simulink model "DriveSimulation"  (R2019b)
settings: Solver=FixedStepAuto  StartTime=0.0  StopTime=inf  FixedStep=dt  RelTol=1e-3
model workspace (MAT data in the model file):
  AcceNoisePower = 0.01
  AcceNoiseStd = 0.1
  AcceTs = 0.01
  ControlTs = 0.1
  GPSNoisePower = 0.001
  GPSNoiseStd = 1
  GPSTs = 0.5
  GyroNoisePower = 0.001
  GyroNoiseStd = 0.000174532925199
  GyroTs = 0.01
  L = 4
  SteeringRange = 0.837758040957
  Ts = 0.01
  Var = 0
  Vmax = 41.6666666667
  dt = 0.01
undefined symbols (not defined in the file): DiscIntNeverNeededParam, m, rad, s
libraries: simulink x6, sim3dlib x1, sim3dautolib x1, aerolibanimutils x1
settings Model: Creator=alons  LastModifiedBy=alons
settings DataIOCC: ReturnWorkspaceOutputs=off
settings DebuggingCC: ArithmeticOperatorsInVariantConditions=warning
settings SFSimCC: CustomCodeUndefinedFunction=UseInterfaceOnly

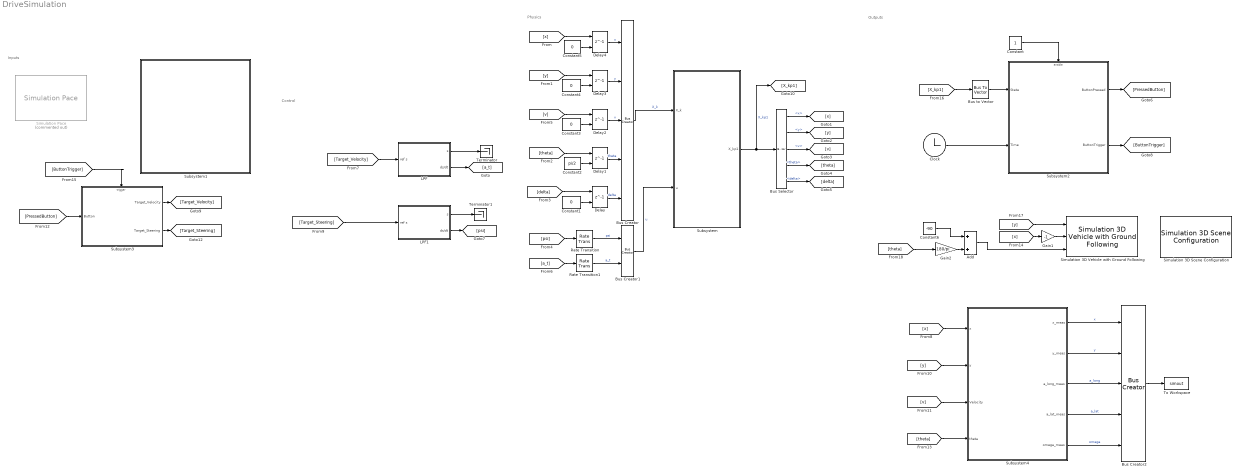
== system DriveSimulation ==
  note: Control
  note: Physics
  note: Inputs
  note: Outputs
  Add : Sum
  Bus Creator : BusCreator  Inputs=5
  Bus Creator1 : BusCreator  Inputs=2
  Bus Creator2 : BusCreator  Inputs=5
  Bus Selector : BusSelector  OutputSignals=x,y,v,theta,delta
  Bus to Vector : BusToVector
  Clock : Clock
  Constant : Constant  SampleTime=0
      settings: OpenFcn=|
      | if get_param(gcbh,'value')-48
      |    set_param(gcbh,'value','0','backgroundcolor','red');
      | else
      |    set_param(gcbh,'value','1','backgroundcolor','green');
      | end
  Constant{1,3..5} (4 alike) : Constant  Value=0
  Constant2 : Constant  Value=pi/2
  Constant6 : Constant  Value=-90
  Delay{,1..4} (5 alike) : Delay  DelayLength=1  InitialConditionSource=Input port
      settings: InputPortMap=u0,p4
  Gain1 : Gain  Gain=-1
  Gain2 : Gain  Gain=180/pi
  LPF : Subsystem  mask{Freq=1, Rate_Max=10 %m/s^2, Rate_Min=-20 %m/s^2}
      mask prompts: Freq "LPF Freq [Hz]"; Rate_Max "Maximum ds/dt slope"; Rate_Min "Minimum ds/dt slope"
      mask Display: fprintf('LPF /w Rate Limit \n%g[Hz]',Freq);
  LPF1 : Subsystem  mask{Freq=2, Rate_Max=20*pi/180 %rad/s, Rate_Min=-20*pi/180 %rad/s}
      mask prompts: Freq "LPF Freq [Hz]"; Rate_Max "Maximum ds/dt slope"; Rate_Min "Minimum ds/dt slope"
      mask Display: fprintf('LPF /w Rate Limit \n%g[Hz]',Freq);
  Rate Transition : RateTransition  OutPortSampleTime=dt
  Rate Transition1 : RateTransition  OutPortSampleTime=dt
  Simulation 3D Scene Configuration : sim3dlib/Simulation 3D Scene Configuration  Priority=0  SceneDesc=Curved road  vehTagList={'Scene Origin';'SimulinkVehicle1'}  vehTag=SimulinkVehicle1  OpVisEn=off  Ts=ControlTs  ProjectFormat=Executable  ProjectName=VehicleSimulation.exe  sensorTag=MainCamera1  sensorId=1  sensorName=MainCamera1  mountLoc=Origin  offsetFlag=off  tmountOffset=[0, 0, 0]  rmountOffset=[0, 0, 0]  HorizontalResolution=1280  VerticalResolution=720  HorizontalFOV=60  mountPoint=[0 0 0]  mountOrientation=[0 0 0]  aMode=3  ID=1
      settings: SourceProductName=Automated Driving Toolbox  SourceProductBaseCode=DR
  Simulation 3D Vehicle with Ground Following : sim3dautolib/Simulation 3D Vehicle with Ground Following  Priority=-1  PassVehMesh=Muscle car  VehColor=Red  InitialPos=[0, 0, 0]  InitialRot=[0, 0, 0]  ActorName=SimulinkVehicle1  SampleTime=-1  ActorType=SimulinkVehicle  ID=1  aMode=3  ActorTag=SimulinkVehicle1  CoordinateScheme=ISO  TransformOutportEnabled=off
      settings: SourceProductName=Automated Driving Toolbox  SourceProductBaseCode=DR
  Simulation Pace : aerolibanimutils/Simulation Pace  Commented=on  SimulationPace=1  SleepMode=Auto  OutputPaceError=off  SampleTime=dt
  Subsystem : Subsystem
      mask Display: fprintf('Rear Axle Bicycle Model\n[Kinematic]')
  Subsystem1 : Subsystem  InitFcn=|  mask{dt=0.01, ControlTs=0.1, AcceTs=0.01, GyroTs=0.01, GPSTs=0.5, AcceNoiseStd=0.1, GyroNoiseStd=0.01*pi/180, GPSNoiseStd=1, L=4, Vmax=150/3.6, SteeringRange=48/180*pi}
      | mdlWks=get_param(bdroot,'ModelWorkspace')
      | par = get_param(gcb,'DialogParameters');
      | fnames = fieldnames(par);
      | for ipar=1:length(fnames)
      |    num=str2num(get_param(gcb,fnames{ipar}));
      |    mdlWks.assignin(fnames{ipar},num);
      | end
      | 
      | clear par fnames ipar num mdlWks;
      mask prompts: dt "Physics Time Sample [s]"; ControlTs "Control Time Sample [s]"; AcceTs "Accelerometer Time Sample [s]"; GyroTs "Gyro Time Sample [s]"; GPSTs "GPS Time Sample [s]"; AcceNoiseStd "Accelerometer Noise std [m/s^2]"; GyroNoiseStd "Gyro Noise std [rad/s]"; GPSNoiseStd "GPS Noise std [m]"; L "Bicycle Length [m]"; Vmax "Maximum Velocity [m/s]"; SteeringRange "Steering Range [rad]"
      mask Display:
      | str=[
      |     'Model Workspace Parameters \n\n\n',...
      |     'Physics Sample dt = %g[s]\n\n',...
      |     'Control Sample ControlTs = %g[s]\n\n',...
      |     'Accelerometer Sample AcceTs = %g[s]\n\n',...
      |     'Gyro Sample GyroTs = %g[s]\n\n',...
      |     'GPS Sample GpsTs = %g[s]\n\n',...
      |     'Accelerometer Noise std = %g[m/s^2]\n\n',...
      |     'Gyro Noise std = %g[rad/s^2]\n\n',...
      |     'GPS Noise std = %g[m]\n\n',...
      |     'Bicycle Length L = %g[m]\n\n',...
      |     'Maximum Velocity Vmax = %g[m/s]\n\n',...
      |     'SteeringRange = %g[rad]\n\n',...
      |     ];
      | fprintf(str,dt,ControlTs,AcceTs,GyroTs,GPSTs,...
      |     AcceNoiseStd,GyroNoiseStd,GPSNoiseStd,L,Vmax,SteeringRange);
  Subsystem2 : Subsystem
      settings: OpenFcn=|
      | UserData = get_param([gcb,'/AnimationSfcn'],'UserData');
      | Fig = UserData.Figure;
      | if ishghandle(Fig,'figure');
      |    %bring to the front:
      |    figure(Fig);
      | end
      mask Display:
      | t=linspace(0,2*pi,20);
      | plot(cos(t),sin(t));
      | 
      | x=[-0.4,-0.4,0.6,-0.4];
      | y=[-0.5,0.5,0,-0.5];
      | plot(x,y)
      | 
      | disp('Drive Simulator')
  Subsystem3 : Subsystem
  Subsystem4 : Subsystem
      mask Display: disp('Sensor Readings')
  Terminator : Terminator
  Terminator1 : Terminator
  To Workspace : ToWorkspace  VariableName=simout  SaveFormat=Timeseries  SampleTime=-1
  wires:
  [psi] -> Rate Transition/1
  [a_t] -> Rate Transition1/1
  Bus Creator/1 -> Subsystem/1(X_k)  "X_k"
  Bus Creator1/1 -> Subsystem/2(u)  "u"
  Constant/1 -> Subsystem2/Enable
  Clock/1 -> Subsystem2/2(Time)
  Bus Selector/2 -> [y]  "<y>"
  Bus Selector/1 -> [x]  "<x>"
  Bus Selector/3 -> [v]  "<v>"
  Bus Selector/5 -> [delta]  "<delta>"
  Bus Selector/4 -> [theta]  "<theta>"
  [Target_Velocity] -> LPF/1(ref s)
  [Target_Steering] -> LPF1/1(ref s)
  LPF1/2(ds/dt) -> [psi]
  [PressedButton] -> Subsystem3/1(Button)
  [ButtonTrigger] -> Subsystem3/Trigger
  Subsystem3/1(Target_Velocity) -> [Target_Velocity]
  Subsystem3/2(Target_Steering) -> [Target_Steering]
  Rate Transition/1 -> Bus Creator1/1  "psi"
  Rate Transition1/1 -> Bus Creator1/2  "a_t"
  [X_kp1] -> Bus to Vector/1
  Bus to Vector/1 -> Subsystem2/1(State)
  Delay/1 -> Bus Creator/5  "delta"
  [delta] -> Delay/1
  Constant1/1 -> Delay/2
  Delay1/1 -> Bus Creator/4  "theta"
  Delay2/1 -> Bus Creator/3  "v"
  Delay3/1 -> Bus Creator/2  "y"
  Delay4/1 -> Bus Creator/1  "x"
  [x] -> Delay4/1
  [v] -> Delay2/1
  [y] -> Delay3/1
  [theta] -> Delay1/1
  Constant2/1 -> Delay1/2
  Constant3/1 -> Delay2/2
  Constant4/1 -> Delay3/2
  Constant5/1 -> Delay4/2
  Subsystem/1(X_kp1) -> [X_kp1], Bus Selector/1  "X_kp1"
  LPF/2(ds/dt) -> [a_t]
  LPF/1(s) -> Terminator/1
  LPF1/1(s) -> Terminator1/1
  Subsystem2/1(ButtonPressed) -> [PressedButton]
  Subsystem2/2(ButtonTrigger) -> [ButtonTrigger]
  [x] -> Subsystem4/1(x)
  [y] -> Subsystem4/2(y)
  [v] -> Subsystem4/3(Velocity)
  [theta] -> Subsystem4/4(theta)
  Subsystem4/5(omega_meas) -> Bus Creator2/5  "omega"
  Subsystem4/4(a_lat_meas) -> Bus Creator2/4  "a_lat"
  Subsystem4/3(a_long_meas) -> Bus Creator2/3  "a_long"
  Subsystem4/2(y_meas) -> Bus Creator2/2  "y"
  Subsystem4/1(x_meas) -> Bus Creator2/1  "x"
  Bus Creator2/1 -> To Workspace/1
  [x] -> Gain1/1
  [theta] -> Gain2/1
  Gain1/1 -> Simulation 3D Vehicle with Ground Following/2
  Gain2/1 -> Add/2
  Add/1 -> Simulation 3D Vehicle with Ground Following/3
  Constant6/1 -> Add/1
  [y] -> Simulation 3D Vehicle with Ground Following/1

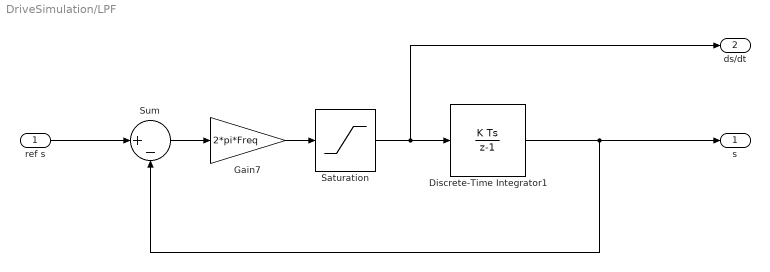
== system DriveSimulation/LPF ==
  ref s : Inport
  Discrete-Time Integrator1 : DiscreteIntegrator  SampleTime=-1  ICPrevOutput=DiscIntNeverNeededParam  ICPrevScaledInput=DiscIntNeverNeededParam
  Gain7 : Gain  Gain=2*pi*Freq
  Saturation : Saturate  UpperLimit=Rate_Max  LowerLimit=Rate_Min
  Sum : Sum  Inputs=|+-
  s : Outport  VectorParamsAs1DForOutWhenUnconnected=off
  ds/dt : Outport  Port=2  VectorParamsAs1DForOutWhenUnconnected=off
  wires:
  Discrete-Time Integrator1/1 -> s/1, Sum/2
  Sum/1 -> Gain7/1
  Gain7/1 -> Saturation/1
  ref s/1 -> Sum/1
  Saturation/1 -> ds/dt/1, Discrete-Time Integrator1/1

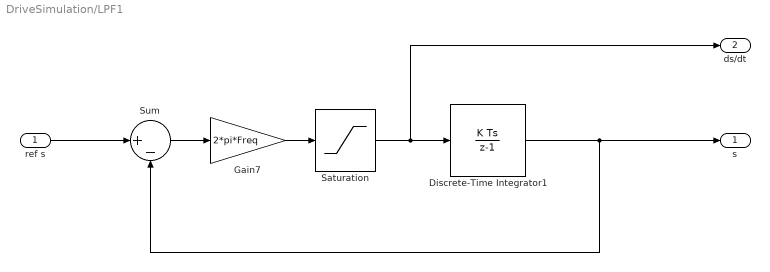
== system DriveSimulation/LPF1 ==
  ref s : Inport
  Discrete-Time Integrator1 : DiscreteIntegrator  SampleTime=-1  ICPrevOutput=DiscIntNeverNeededParam  ICPrevScaledInput=DiscIntNeverNeededParam
  Gain7 : Gain  Gain=2*pi*Freq
  Saturation : Saturate  UpperLimit=Rate_Max  LowerLimit=Rate_Min
  Sum : Sum  Inputs=|+-
  s : Outport  VectorParamsAs1DForOutWhenUnconnected=off
  ds/dt : Outport  Port=2  VectorParamsAs1DForOutWhenUnconnected=off
  wires:
  Discrete-Time Integrator1/1 -> s/1, Sum/2
  Sum/1 -> Gain7/1
  Gain7/1 -> Saturation/1
  ref s/1 -> Sum/1
  Saturation/1 -> ds/dt/1, Discrete-Time Integrator1/1

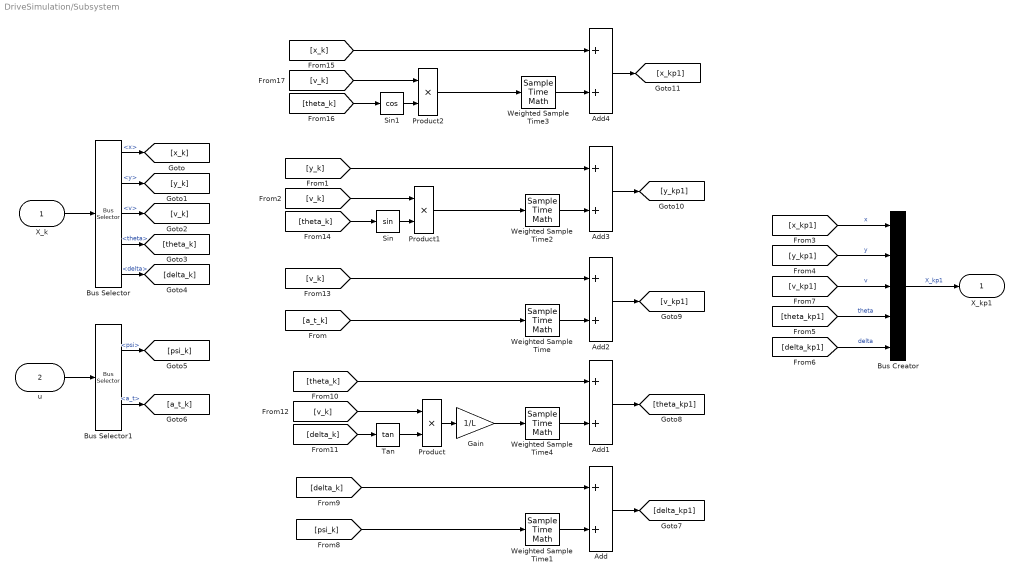
== system DriveSimulation/Subsystem ==
  X_k : Inport
  u : Inport  Port=2
  Add{,1..4} (5 alike) : Sum
  Bus Creator : BusCreator  Inputs=5
  Bus Selector : BusSelector  OutputSignals=x,y,v,theta,delta
  Bus Selector1 : BusSelector  OutputSignals=psi,a_t
  Gain : Gain  Gain=1/L
  Product : Product
  Product1 : Product
  Product2 : Product
  Sin : Trigonometry
  Sin1 : Trigonometry  Operator=cos
  Tan : Trigonometry  Operator=tan
  Weighted Sample Time{,1..4} (5 alike) : SampleTimeMath  TsampMathOp=*
  X_kp1 : Outport  VectorParamsAs1DForOutWhenUnconnected=off
  wires:
  X_k/1 -> Bus Selector/1
  Bus Selector/1 -> [x_k]  "<x>"
  Bus Selector/2 -> [y_k]  "<y>"
  Bus Selector/3 -> [v_k]  "<v>"
  Bus Selector/4 -> [theta_k]  "<theta>"
  Bus Selector/5 -> [delta_k]  "<delta>"
  u/1 -> Bus Selector1/1
  Bus Selector1/1 -> [psi_k]  "<psi>"
  Bus Selector1/2 -> [a_t_k]  "<a_t>"
  [a_t_k] -> Weighted Sample Time/1
  [y_kp1] -> Bus Creator/2  "y"
  Bus Creator/1 -> X_kp1/1  "X_kp1"
  [theta_kp1] -> Bus Creator/4  "theta"
  [x_kp1] -> Bus Creator/1  "x"
  [v_kp1] -> Bus Creator/3  "v"
  [delta_kp1] -> Bus Creator/5  "delta"
  [psi_k] -> Weighted Sample Time1/1
  Weighted Sample Time1/1 -> Add/2
  [delta_k] -> Add/1
  Add/1 -> [delta_kp1]
  Add1/1 -> [theta_kp1]
  [theta_k] -> Add1/1
  [delta_k] -> Tan/1
  Tan/1 -> Product/2
  [v_k] -> Product/1
  Gain/1 -> Weighted Sample Time4/1
  Product/1 -> Gain/1
  Add2/1 -> [v_kp1]
  Weighted Sample Time/1 -> Add2/2
  [v_k] -> Add2/1
  Add3/1 -> [y_kp1]
  [y_k] -> Add3/1
  Product1/1 -> Weighted Sample Time2/1
  [v_k] -> Product1/1
  Sin/1 -> Product1/2
  [theta_k] -> Sin/1
  Add4/1 -> [x_kp1]
  Sin1/1 -> Product2/2
  [v_k] -> Product2/1
  [x_k] -> Add4/1
  [theta_k] -> Sin1/1
  Product2/1 -> Weighted Sample Time3/1
  Weighted Sample Time2/1 -> Add3/2
  Weighted Sample Time3/1 -> Add4/2
  Weighted Sample Time4/1 -> Add1/2

== system DriveSimulation/Subsystem1 ==

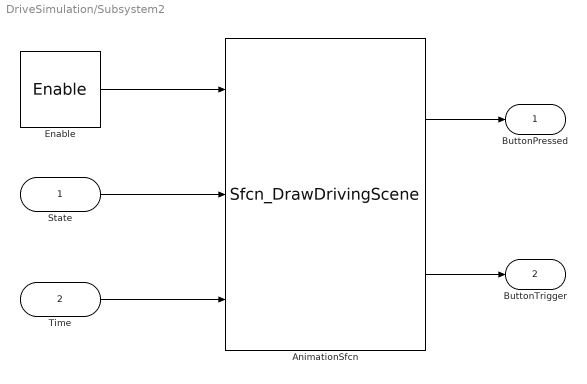
== system DriveSimulation/Subsystem2 ==
  State : Inport
  Time : Inport  Port=2
  Enable : EnablePort  StatesWhenEnabling=reset  ShowOutputPort=on
  AnimationSfcn : M-S-Function  FunctionName=Sfcn_DrawDrivingScene  Parameters=ControlTs,L,Vmax
  ButtonPressed : Outport  VectorParamsAs1DForOutWhenUnconnected=off
  ButtonTrigger : Outport  Port=2  VectorParamsAs1DForOutWhenUnconnected=off
  wires:
  State/1 -> AnimationSfcn/2
  Enable/1 -> AnimationSfcn/1
  AnimationSfcn/1 -> ButtonPressed/1
  AnimationSfcn/2 -> ButtonTrigger/1
  Time/1 -> AnimationSfcn/3

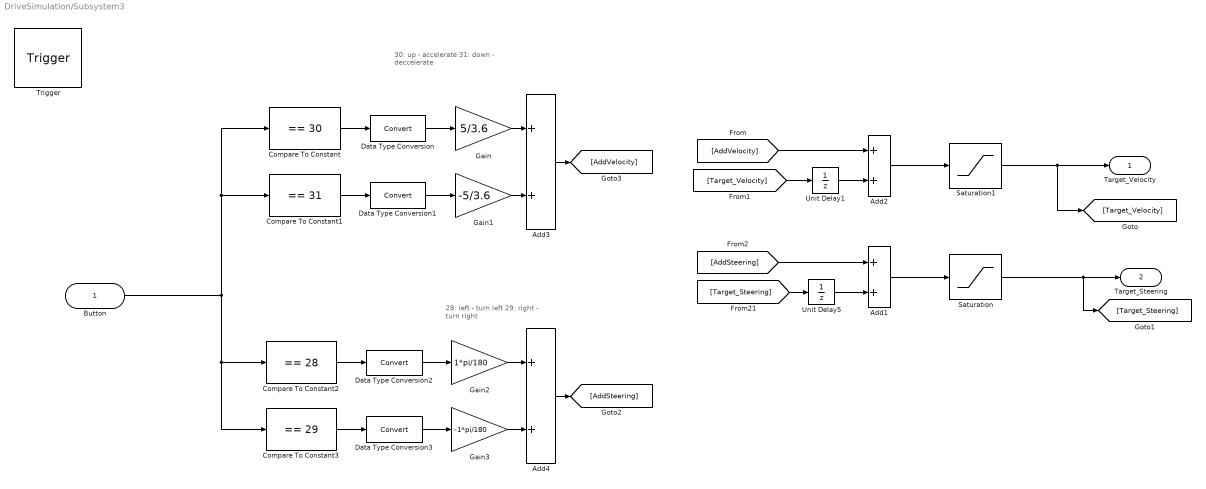
== system DriveSimulation/Subsystem3 ==
  note: 30: up - accelerate
      | 31: down - deccelerate
  note: 28: left - turn left
      | 29: right - turn right
  Button : Inport
  Trigger : TriggerPort  VariantControl=Variant  PortDimensions=1
  Add{1..4} (4 alike) : Sum
  Compare To Constant : simulink/Logic and Bit Operations/Compare To Constant  relop===  const=30  OutDataTypeStr=boolean
  Compare To Constant1 : simulink/Logic and Bit Operations/Compare To Constant  relop===  const=31  OutDataTypeStr=boolean
  Compare To Constant2 : simulink/Logic and Bit Operations/Compare To Constant  relop===  const=28  OutDataTypeStr=boolean
  Compare To Constant3 : simulink/Logic and Bit Operations/Compare To Constant  relop===  const=29  OutDataTypeStr=boolean
  Data Type Conversion{,1..3} (4 alike) : DataTypeConversion
  Gain : Gain  Gain=5/3.6
  Gain1 : Gain  Gain=-5/3.6
  Gain2 : Gain  Gain=1*pi/180
  Gain3 : Gain  Gain=-1*pi/180
  Saturation : Saturate  UpperLimit=SteeringRange/2  LowerLimit=-SteeringRange/2
  Saturation1 : Saturate  UpperLimit=Vmax  LowerLimit=0
  Unit Delay1 : UnitDelay  SampleTime=-1  HasFrameUpgradeWarning=on
  Unit Delay5 : UnitDelay  SampleTime=-1  HasFrameUpgradeWarning=on
  Target_Velocity : Outport  VectorParamsAs1DForOutWhenUnconnected=off
  Target_Steering : Outport  Port=2  VectorParamsAs1DForOutWhenUnconnected=off
  wires:
  [Target_Velocity] -> Unit Delay1/1
  Unit Delay1/1 -> Add2/2
  Add2/1 -> Saturation1/1
  [AddVelocity] -> Add2/1
  Add1/1 -> Saturation/1
  [Target_Steering] -> Unit Delay5/1
  Unit Delay5/1 -> Add1/2
  [AddSteering] -> Add1/1
  Add4/1 -> [AddSteering]
  Compare To Constant/1 -> Data Type Conversion/1
  Data Type Conversion/1 -> Gain/1
  Button/1 -> Compare To Constant1/1, Compare To Constant/1, Compare To Constant3/1, Compare To Constant2/1
  Compare To Constant1/1 -> Data Type Conversion1/1
  Data Type Conversion1/1 -> Gain1/1
  Gain1/1 -> Add3/2
  Gain/1 -> Add3/1
  Add3/1 -> [AddVelocity]
  Data Type Conversion2/1 -> Gain2/1
  Compare To Constant2/1 -> Data Type Conversion2/1
  Data Type Conversion3/1 -> Gain3/1
  Compare To Constant3/1 -> Data Type Conversion3/1
  Gain2/1 -> Add4/1
  Gain3/1 -> Add4/2
  Saturation1/1 -> [Target_Velocity], Target_Velocity/1
  Saturation/1 -> [Target_Steering], Target_Steering/1

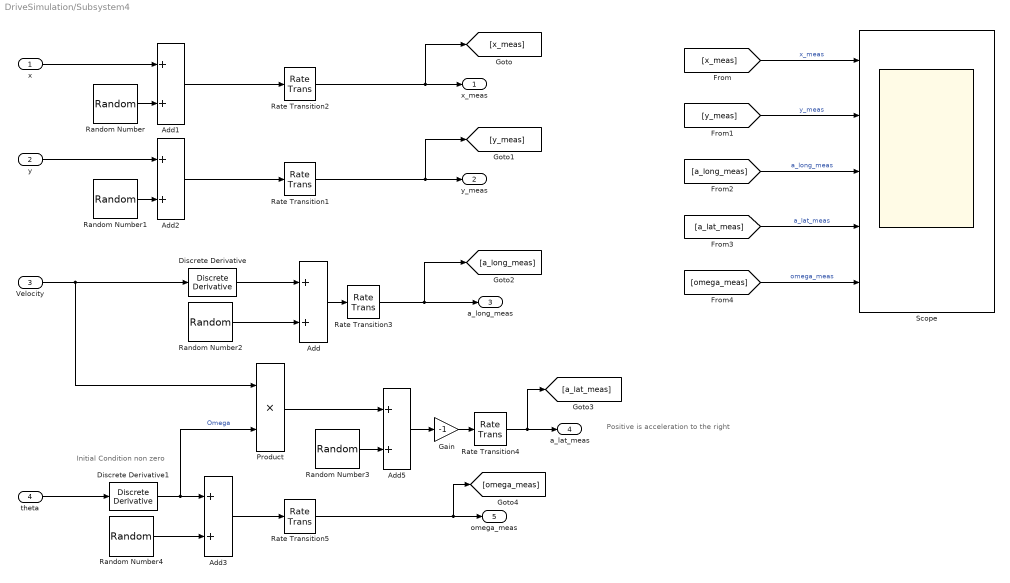
== system DriveSimulation/Subsystem4 ==
  note: Initial Condition non zero
  note: Positive is acceleration to the right
  x : Inport
  y : Inport  Port=2
  Velocity : Inport  Port=3
  theta : Inport  Port=4
  Add{,1..3,5} (5 alike) : Sum
  Discrete Derivative : simulink/Discrete/Discrete Derivative  gainval=1.0  ICPrevScaledInput=0.0  OutMin=[]  OutMax=[]  OutDataType=fixdt(1, 16)  OutScaling=2^-10  DoSatur=off
  Discrete Derivative1 : simulink/Discrete/Discrete Derivative  gainval=1.0  ICPrevScaledInput=pi/2/dt  OutMin=[]  OutMax=[]  OutDataType=fixdt(1, 16)  OutScaling=2^-10  DoSatur=off
  Gain : Gain  Gain=-1
  Product : Product
  Random Number : RandomNumber  Variance=(GPSNoiseStd^2)
  Random Number1 : RandomNumber  Variance=(GPSNoiseStd^2)  Seed=2
  Random Number2 : RandomNumber  Variance=AcceNoiseStd^2  Seed=3
  Random Number3 : RandomNumber  Variance=AcceNoiseStd^2  Seed=4
  Random Number4 : RandomNumber  Variance=GyroNoiseStd  Seed=5
  Rate Transition1 : RateTransition  OutPortSampleTime=GPSTs
  Rate Transition2 : RateTransition  OutPortSampleTime=GPSTs
  Rate Transition3 : RateTransition  OutPortSampleTime=AcceTs
  Rate Transition4 : RateTransition  OutPortSampleTime=AcceTs
  Rate Transition5 : RateTransition  OutPortSampleTime=GyroTs
  Scope : Scope  NumInputPorts=5
  x_meas : Outport  VectorParamsAs1DForOutWhenUnconnected=off
  y_meas : Outport  Port=2  VectorParamsAs1DForOutWhenUnconnected=off
  a_long_meas : Outport  Port=3  VectorParamsAs1DForOutWhenUnconnected=off
  a_lat_meas : Outport  Port=4  VectorParamsAs1DForOutWhenUnconnected=off
  omega_meas : Outport  Port=5  VectorParamsAs1DForOutWhenUnconnected=off
  wires:
  Random Number/1 -> Add1/2
  Random Number2/1 -> Add/2
  Random Number3/1 -> Add5/2
  Random Number1/1 -> Add2/2
  Velocity/1 -> Product/1, Discrete Derivative/1
  Discrete Derivative1/1 -> Product/2, Add3/1  "Omega"
  Product/1 -> Add5/1
  y/1 -> Add2/1
  Random Number4/1 -> Add3/2
  Add1/1 -> Rate Transition2/1
  Add/1 -> Rate Transition3/1
  Add3/1 -> Rate Transition5/1
  Add2/1 -> Rate Transition1/1
  x/1 -> Add1/1
  Add5/1 -> Gain/1
  theta/1 -> Discrete Derivative1/1
  Gain/1 -> Rate Transition4/1
  [x_meas] -> Scope/1  "x_meas"
  [y_meas] -> Scope/2  "y_meas"
  [a_long_meas] -> Scope/3  "a_long_meas"
  [a_lat_meas] -> Scope/4  "a_lat_meas"
  [omega_meas] -> Scope/5  "omega_meas"
  Rate Transition2/1 -> [x_meas], x_meas/1
  Rate Transition1/1 -> [y_meas], y_meas/1
  Rate Transition3/1 -> [a_long_meas], a_long_meas/1
  Rate Transition4/1 -> [a_lat_meas], a_lat_meas/1
  Rate Transition5/1 -> [omega_meas], omega_meas/1
  Discrete Derivative/1 -> Add/1
